simulink model "a8"  (R2021a)
settings: Solver=VariableStepAuto  StartTime=0.0  StopTime=3  RelTol=1e-3
undefined symbols (not defined in the file or in its folder): Down, Ion, Lithium, Up
libraries: spsCurrentMeasurementLib x22, spsVoltageMeasurementLib x17, spsSeriesRLCBranchLib x11, spsGroundLib x6, powerlib_extras x4, spsACVoltageSourceLib x3, spsIGBTDiodeLib x3, dspsigops x3, spsPower3phInstantaneousLib x3, spsDiodeLib x2, spsUniversalBridgeLib x2, spsBatteryLib x1
(part 2 of 2)

== matlab function a8/PnO MPPT ==
  settings: updateMethod=DISCRETE
  data: v input; d output; i input
function d = fcn(v,i)
persistent vprev;
persistent dprev;
persistent pprev;


   if isempty(vprev)
       vprev=0;
   end
   if isempty(dprev)
       dprev=0;
   end
   if isempty(pprev)
       pprev=0;
   end

   d = dprev;
   p = v*i;
   deltav = v - vprev;
   deltap = p -pprev;
   if deltap>0
       if deltav>0
           d = dprev - 0.05;
       elseif deltav <0
           d = dprev+0.05;
       end
   elseif deltap<0
       if deltav>0
           d = dprev+0.05;
       elseif deltav<0
           d = dprev-0.05;
       end
   end


   if d>0.9
       d=0.9;
   elseif d<0
       d=0;
   end
   vprev = v;
   pprev = p;
   dprev = d;
